simulink model "hierchical_control"  (R2023b)
settings: Solver=VariableStepAuto  StartTime=0.0  StopTime=tot_time  RelTol=1e-3
InitFcn:
  | addpath('TRAJECTORIES\');
  | %square_coplanar
  | circular_coplanar
StartFcn:
  | %% Setup Video e Timer
  | videoFile = 'Hierarchical_quad.avi';
  | %videoFile = 'Hierarchical_circ.avi';
  | videoObj = VideoWriter(videoFile);
  | videoObj.FrameRate = 30;
  | open(videoObj);
  | assignin('base','videoObj',videoObj);
  | 
  | 
  | t = timer('ExecutionMode','fixedSpacing','Period',0.05,'StartDelay',2,...
  |           'TimerFcn',@(~,~) captureFrame(findall(0,'Type','figure','Name','UAV Animation'), videoObj));
  | start(t);
  | 
  | 
  | assignin('base','videoTimer',t);
StopFcn:
  | % Default graphics settings
  | set(0, 'DefaultTextInterpreter', 'latex')
  | set(0, 'DefaultLegendInterpreter', 'latex')
  | set(0, 'DefaultAxesTickLabelInterpreter', 'latex')
  | lw = 2;
  | 
  | plot_errors = figure('Renderer', 'painters', 'Position', [10 10 900 650]);
  | 
  | subplot(2,1,1)
  | plot(out.tout, out.err_p.signals.values(1,:), 'k-', 'Linewidth', lw ,'Color', [0.2, 0.2, 0.2]);
  | hold on
  | plot(out.tout, out.err_p.signals.values(2,:), 'k-', 'Linewidth', lw ,'Color', [1, 0, 0]);
  | hold on
  | plot(out.tout, out.err_p.signals.values(3,:), 'k-', 'Linewidth', lw ,'Color', [0, 0, 1]);
  | 
  | legend({'x-axis', 'y-axis', 'z-axis'}, ...
  |        'Location', 'northeast', ...
  |        'Orientation', 'vertical', ...
  |        'FontSize', 16);
  | 
  | 
  | %xlabel('Time [s]')
  | ylabel('$e_p$ [m]')
  | 
  | set(gca, 'FontSize',20);
  | 
  | %Grid
  | grid on
  | box on
  | 
  | 
  | %----------------------------------------------------------
  | 
  | subplot(2,1,2)
  | plot(out.tout, out.dot_err_p.signals.values(1,:), 'k-', 'Linewidth', lw ,'Color', [0.2, 0.2, 0.2]);
  | hold on
  | plot(out.tout, out.dot_err_p.signals.values(2,:), 'k-', 'Linewidth', lw ,'Color', [1, 0, 0]);
  | hold on
  | plot(out.tout, out.dot_err_p.signals.values(3,:), 'k-', 'Linewidth', lw ,'Color', [0, 0, 1]);
  | 
  | legend({'x-axis', 'y-axis', 'z-axis'}, ...
  |        'Location', 'southeast', ...
  |        'Orientation', 'vertical', ...
  |        'FontSize', 16);
  | 
  | 
  | xlabel('Time [s]')
  | ylabel('$\dot{e}_p$ [m/s]')
  | 
  | set(gca, 'FontSize',20);
  | 
  | %Grid
  | grid on
  | box on
  | 
  | %Options
  | set(gcf,'color','w');
  | set(plot_errors, 'MenuBar', 'none', 'ToolBar', 'none');
  | 
  | exportgraphics(plot_errors, 'Hierarchical_lin_err.pdf');
  | 
  | %--------------------------------------------------
  | plot_errors_or = figure('Renderer', 'painters', 'Position', [10 10 900 650]);
  | 
  | subplot(2,1,1)
  | plot(out.tout, out.err_eta.signals.values(1,:), 'k-', 'Linewidth', lw ,'Color', [0.2, 0.2, 0.2]);
  | hold on
  | plot(out.tout, out.err_eta.signals.values(2,:), 'k-', 'Linewidth', lw ,'Color', [1, 0, 0]);
  | hold on
  | plot(out.tout, out.err_eta.signals.values(3,:), 'k-', 'Linewidth', lw ,'Color', [0, 0, 1]);
  | 
  | legend({'x-axis', 'y-axis', 'z-axis'}, ...
  |        'Location', 'southeast', ...
  |        'Orientation', 'vertical', ...
  |        'FontSize', 16);
  | 
  | 
  | ylabel('$e_{\eta}$ [rad]')
  | 
  | set(gca, 'FontSize',20);
  | 
  | %Grid
  | grid on
  | box on
  | 
  | 
  | %----------------------------------------------------------
  | 
  | subplot(2,1,2)
  | plot(out.tout, out.dot_err_eta.signals.values(1,:), 'k-', 'Linewidth', lw ,'Color', [0.2, 0.2, 0.2]);
  | hold on
  | plot(out.tout, out.dot_err_eta.signals.values(2,:), 'k-', 'Linewidth', lw ,'Color', [1, 0, 0]);
  | hold on
  | plot(out.tout, out.dot_err_eta.signals.values(3,:), 'k-', 'Linewidth', lw ,'Color', [0, 0, 1]);
  | 
  | legend({'x-axis', 'y-axis', 'z-axis'}, ...
  |        'Location', 'southeast', ...
  |        'Orientation', 'vertical', ...
  |        'FontSize', 16);
  | 
  | xlabel('Time [s]')
  | ylabel('$\dot{e_{\eta}}$ [rad/s]')
  | 
  | set(gca, 'FontSize',20);
  | 
  | %Grid
  | grid on
  | box on
  | 
  | %Options
  | set(gcf,'color','w');
  | set(plot_errors_or, 'MenuBar', 'none', 'ToolBar', 'none');
  | 
  | exportgraphics(plot_errors_or, 'Hierarchical_or_err.pdf');
  | 
  | 
  | %--------------------------------------------------------------
  | plot_pos_or = figure('Renderer', 'painters', 'Position', [10 10 900 650]);
  | 
  | subplot(2,1,1)
  | plot(out.tout, out.position.signals.values(1,:), 'k-', 'Linewidth', lw ,'Color', [0.2, 0.2, 0.2]);
  | hold on
  | plot(out.tout, out.position.signals.values(2,:), 'k-', 'Linewidth', lw ,'Color', [1, 0, 0]);
  | 
  | legend({'x-axis', 'y-axis'}, ...
  |        'Location', 'southeast', ...
  |        'Orientation', 'vertical', ...
  |        'FontSize', 16);
  | 
  | 
  | ylabel('$x,y$ [m]')
  | 
  | set(gca, 'FontSize',20);
  | 
  | %Grid
  | grid on
  | box on
  | 
  | 
  | %----------------------------------------------------------
  | 
  | subplot(2,1,2)
  | plot(out.tout, out.orientation.signals.values(1,:), 'k-', 'Linewidth', lw ,'Color', [0.2, 0.2, 0.2]);
  | hold on
  | plot(out.tout, out.orientation.signals.values(2,:), 'k-', 'Linewidth', lw ,'Color', [1, 0, 0]);
  | 
  | legend({'x-axis', 'y-axis'}, ...
  |        'Location', 'southeast', ...
  |        'Orientation', 'vertical', ...
  |        'FontSize', 16);
  | 
  | xlabel('Time [s]')
  | ylabel('$\phi,\theta$ [rad]')
  | 
  | set(gca, 'FontSize',20);
  | 
  | %Grid
  | grid on
  | box on
  | 
  | %Options
  | set(gcf,'color','w');
  | set(plot_pos_or, 'MenuBar', 'none', 'ToolBar', 'none');
  | 
  | exportgraphics(plot_pos_or, 'Hierarchical_pos_or.pdf');
  | 
  | %----------------------------------------------------------------------------------
  | 
  | plot_uT = figure('Renderer', 'painters', 'Position', [10 10 900 300]);
  | 
  | plot(out.tout, out.uT.signals.values, 'k-', 'Linewidth', lw ,'Color', [0.2, 0.2, 0.2]);
  | 
  | ylabel('$u_T$ [N]')
  | xlabel('Time [s]')
  | 
  | 
  | set(gca, 'FontSize',20);
  | 
  | %Grid
  | grid on
  | box on
  | 
  | %Options
  | set(gcf,'color','w');
  | set(plot_pos_or, 'MenuBar', 'none', 'ToolBar', 'none');
  | 
  | exportgraphics(plot_uT, 'Hierarchical_uT.pdf');
  | 
  | 
  | 
  | %---------------------------------------------------------------------
  | 
  | 
  | videoObj = evalin('base','videoObj');
  | t = evalin('base','videoTimer');
  | 
  | 
  | stop(t);
  | delete(t);
  | close(videoObj);
  | 
  | 
  | clear videoObj videoTimer
  | disp('Saved Video UAV');
undefined symbols (not defined in the file or in its folder): Ib, lin_vel_0, mass, Ts
libraries: robotcorelib x2, uavutilslib x1
settings Model: Creator=fabioruggiero  LastModifiedBy=laura
settings ModelReferenceCC: EnableRefExpFcnMdlSchedulingChecks=on

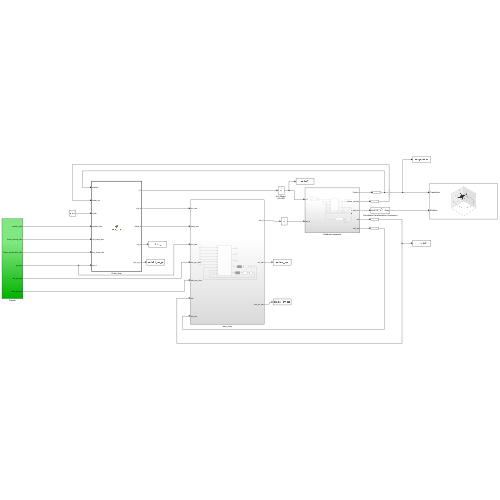
[thumbnail: Simulink's stored preview of the top-level diagram]
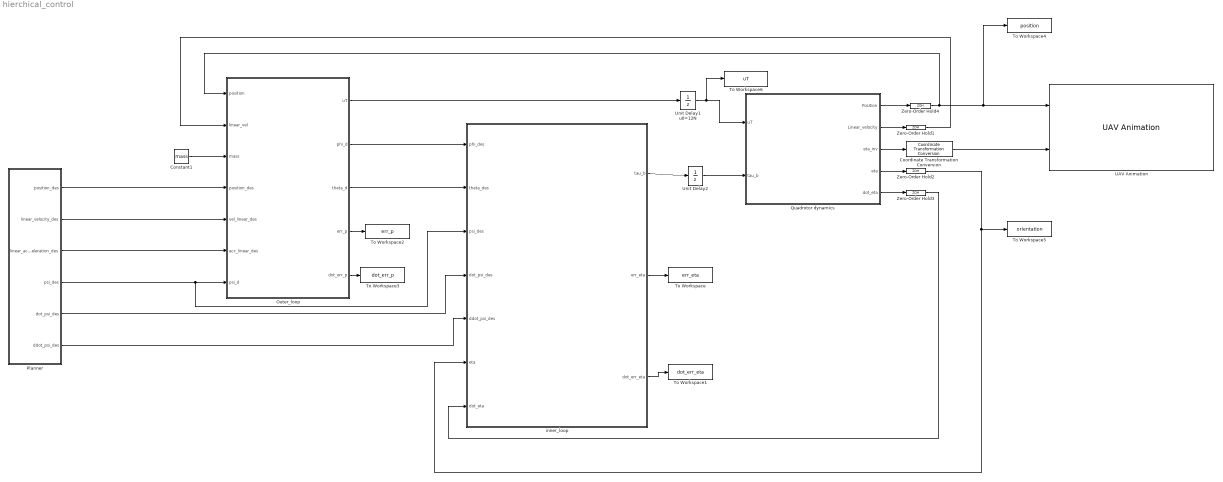
== system hierchical_control ==
  Constant1 : Constant  Value=mass
  Coordinate Transformation Conversion : robotcorelib/Coordinate Transformation Conversion  InputRepresentation=Euler Angles  InputEulerSequence=ZYX  ShowTrVecInputPort=on  OutputRepresentation=Quaternion  OutputEulerSequence=ZYX  ShowTrVecOutputPort=on  SimulateUsing=Interpreted execution
  Outer_loop : MATLAB Function  TreatAsAtomicUnit=on
  Planner : Subsystem
  Quadrotor dynamics : Subsystem
  To Workspace : ToWorkspace  VariableName=err_eta  SaveFormat=Structure With Time  SampleTime=-1
  To Workspace1 : ToWorkspace  VariableName=dot_err_eta  SaveFormat=Structure With Time  SampleTime=-1
  To Workspace2 : ToWorkspace  VariableName=err_p  SaveFormat=Structure With Time  SampleTime=-1
  To Workspace3 : ToWorkspace  VariableName=dot_err_p  SaveFormat=Structure With Time  SampleTime=-1
  To Workspace4 : ToWorkspace  VariableName=position  SaveFormat=Structure With Time  SampleTime=-1
  To Workspace5 : ToWorkspace  VariableName=orientation  SaveFormat=Structure With Time  SampleTime=-1
  To Workspace6 : ToWorkspace  VariableName=uT  SaveFormat=Structure With Time  SampleTime=-1
  UAV Animation : uavutilslib/UAV Animation  UAVType=Multirotor  UAVSize=1  InertialZDirection=Down  SampleTime=0.01
  Unit Delay1 u0=12N : UnitDelay  InitialCondition=12  SampleTime=Ts
  Unit Delay2 : UnitDelay  InitialCondition=[0 0 0]'  SampleTime=Ts
  Zero-Order Hold{1..4} (4 alike) : ZeroOrderHold  SampleTime=Ts
  inner_loop : Subsystem
  wires:
  Planner/1(position_des) -> Outer_loop/4(position_des)
  Planner/2(linear_velocity_des) -> Outer_loop/5(vel_linear_des)
  Planner/3(linear_acceleration_des) -> Outer_loop/6(acc_linear_des)
  Planner/4(psi_des) -> Outer_loop/7(psi_d), inner_loop/3(psi_des)
  Constant1/1 -> Outer_loop/3(mass)
  Planner/5(dot_psi_des) -> inner_loop/4(dot_psi_des)
  Planner/6(ddot_psi_des) -> inner_loop/5(ddot_psi_des)
  Outer_loop/1(uT) -> Unit Delay1 u0=12N/1
  Unit Delay1 u0=12N/1 -> To Workspace6/1, Quadrotor dynamics/1(uT)
  inner_loop/1(tau_b) -> Unit Delay2/1
  Unit Delay2/1 -> Quadrotor dynamics/2(tau_b)
  Quadrotor dynamics/1(Position) -> Zero-Order Hold4/1
  Quadrotor dynamics/2(Linear_velocity) -> Zero-Order Hold1/1
  Quadrotor dynamics/3(eta_inv) -> Coordinate Transformation Conversion/1
  Zero-Order Hold4/1 -> To Workspace4/1, UAV Animation/1, Outer_loop/1(position)
  Coordinate Transformation Conversion/1 -> UAV Animation/2
  Zero-Order Hold1/1 -> Outer_loop/2(linear_vel)
  inner_loop/2(err_eta) -> To Workspace/1
  inner_loop/3(dot_err_eta) -> To Workspace1/1
  Outer_loop/4(err_p) -> To Workspace2/1
  Outer_loop/5(dot_err_p) -> To Workspace3/1
  Quadrotor dynamics/5(dot_eta) -> Zero-Order Hold3/1
  Quadrotor dynamics/4(eta) -> Zero-Order Hold2/1
  Zero-Order Hold2/1 -> To Workspace5/1, inner_loop/6(eta)
  Zero-Order Hold3/1 -> inner_loop/7(dot_eta)
  Outer_loop/3(theta_d) -> inner_loop/2(theta_des)
  Outer_loop/2(phi_d) -> inner_loop/1(phi_des)

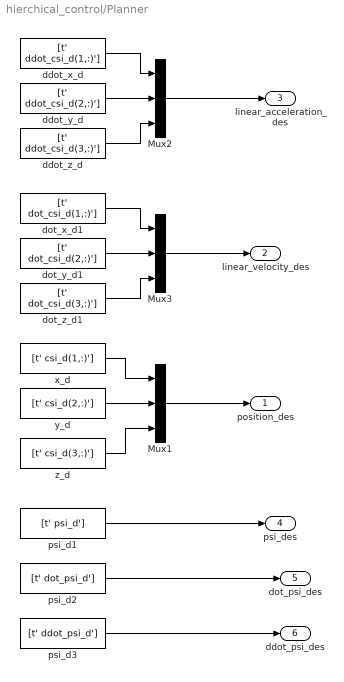
== system hierchical_control/Planner ==
  Mux1 : Mux  Inputs=3
  Mux2 : Mux  Inputs=3
  Mux3 : Mux  Inputs=3
  ddot_x_d : FromWorkspace  VariableName=[t' ddot_csi_d(1,:)']  SampleTime=Ts
  ddot_y_d : FromWorkspace  VariableName=[t' ddot_csi_d(2,:)']  SampleTime=Ts
  ddot_z_d : FromWorkspace  VariableName=[t' ddot_csi_d(3,:)']  SampleTime=Ts
  dot_x_d1 : FromWorkspace  VariableName=[t' dot_csi_d(1,:)']  SampleTime=Ts
  dot_y_d1 : FromWorkspace  VariableName=[t' dot_csi_d(2,:)']  SampleTime=Ts
  dot_z_d1 : FromWorkspace  VariableName=[t' dot_csi_d(3,:)']  SampleTime=Ts
  psi_d1 : FromWorkspace  VariableName=[t' psi_d']  SampleTime=Ts
  psi_d2 : FromWorkspace  VariableName=[t' dot_psi_d']  SampleTime=Ts
  psi_d3 : FromWorkspace  VariableName=[t' ddot_psi_d']  SampleTime=Ts
  x_d : FromWorkspace  VariableName=[t' csi_d(1,:)']  SampleTime=Ts
  y_d : FromWorkspace  VariableName=[t' csi_d(2,:)']  SampleTime=Ts
  z_d : FromWorkspace  VariableName=[t' csi_d(3,:)']  SampleTime=Ts
  position_des : Outport
  linear_velocity_des : Outport  Port=2
  linear_acceleration_des : Outport  Port=3
  psi_des : Outport  Port=4
  dot_psi_des : Outport  Port=5
  ddot_psi_des : Outport  Port=6
  wires:
  y_d/1 -> Mux1/2
  z_d/1 -> Mux1/3
  x_d/1 -> Mux1/1
  ddot_y_d/1 -> Mux2/2
  ddot_z_d/1 -> Mux2/3
  ddot_x_d/1 -> Mux2/1
  Mux2/1 -> linear_acceleration_des/1
  Mux1/1 -> position_des/1
  dot_y_d1/1 -> Mux3/2
  dot_z_d1/1 -> Mux3/3
  dot_x_d1/1 -> Mux3/1
  Mux3/1 -> linear_velocity_des/1
  psi_d1/1 -> psi_des/1
  psi_d3/1 -> ddot_psi_des/1
  psi_d2/1 -> dot_psi_des/1

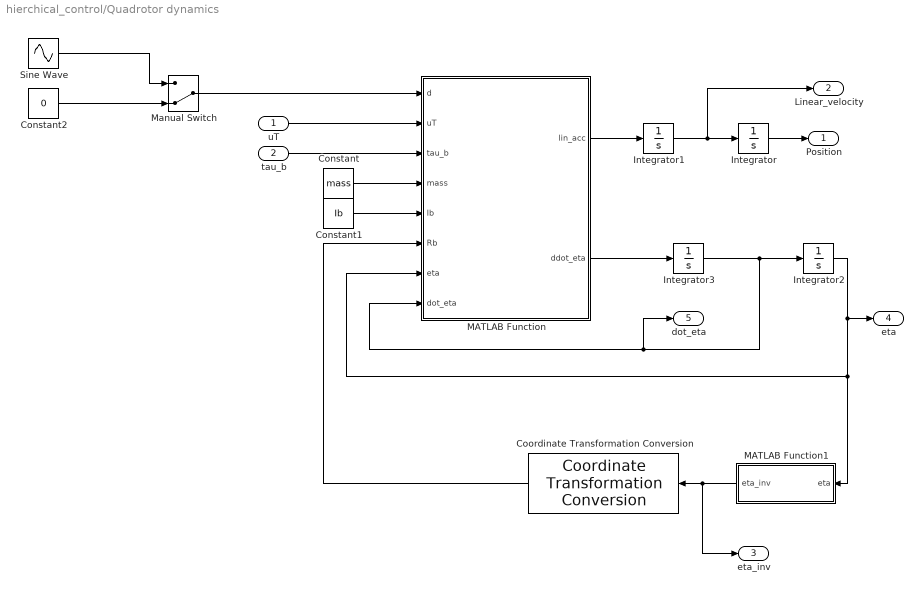
== system hierchical_control/Quadrotor dynamics ==
  uT : Inport
  tau_b : Inport  Port=2
  Constant : Constant  Value=mass
  Constant1 : Constant  Value=Ib
  Constant2 : Constant  Value=0
  Coordinate Transformation Conversion : robotcorelib/Coordinate Transformation Conversion  InputRepresentation=Euler Angles  InputEulerSequence=ZYX  ShowTrVecInputPort=on  OutputRepresentation=Rotation Matrix  OutputEulerSequence=ZYX  ShowTrVecOutputPort=on  SimulateUsing=Interpreted execution
  Integrator : Integrator  InitialCondition=[0 0 -1]'
  Integrator1 : Integrator  InitialCondition=lin_vel_0'
  Integrator2 : Integrator  InitialCondition=[0,0,0]'
  Integrator3 : Integrator  InitialCondition=[0 0 0]'
  MATLAB Function : MATLAB Function  TreatAsAtomicUnit=on
  MATLAB Function1 : MATLAB Function  TreatAsAtomicUnit=on
  Manual Switch : ManualSwitch  CurrentSetting=0
  Sine Wave : Sin  Frequency=0.2  SampleTime=0
  Position : Outport
  Linear_velocity : Outport  Port=2
  eta_inv : Outport  Port=3
  eta : Outport  Port=4
  dot_eta : Outport  Port=5
  wires:
  tau_b/1 -> MATLAB Function/3(tau_b)
  Integrator/1 -> Position/1
  MATLAB Function/1(lin_acc) -> Integrator1/1
  uT/1 -> MATLAB Function/2(uT)
  Integrator1/1 -> Integrator/1, Linear_velocity/1
  Integrator3/1 -> Integrator2/1, dot_eta/1, MATLAB Function/8(dot_eta)
  MATLAB Function/2(ddot_eta) -> Integrator3/1
  Constant/1 -> MATLAB Function/4(mass)
  Constant1/1 -> MATLAB Function/5(Ib)
  Integrator2/1 -> MATLAB Function1/1(eta), MATLAB Function/7(eta), eta/1
  MATLAB Function1/1(eta_inv) -> eta_inv/1, Coordinate Transformation Conversion/1
  Coordinate Transformation Conversion/1 -> MATLAB Function/6(Rb)
  Sine Wave/1 -> Manual Switch/1
  Constant2/1 -> Manual Switch/2
  Manual Switch/1 -> MATLAB Function/1(d)

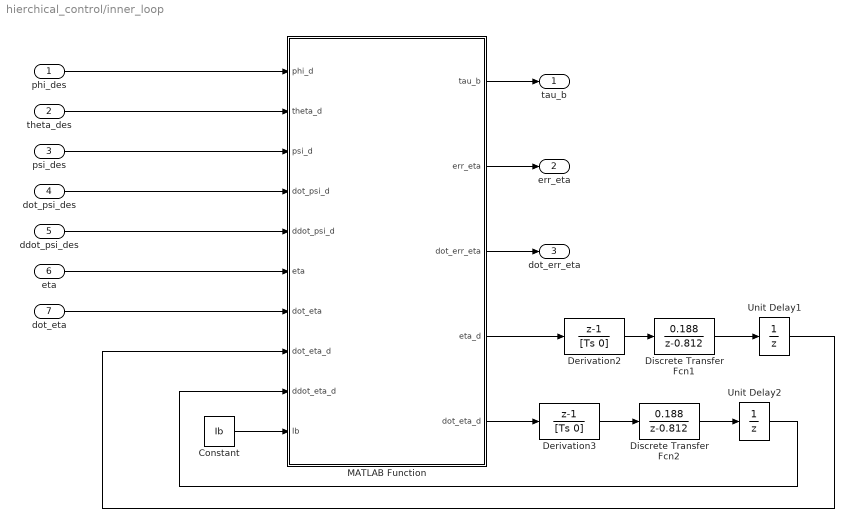
== system hierchical_control/inner_loop ==
  phi_des : Inport
  theta_des : Inport  Port=2
  psi_des : Inport  Port=3
  dot_psi_des : Inport  Port=4
  ddot_psi_des : Inport  Port=5
  eta : Inport  Port=6
  dot_eta : Inport  Port=7
  Constant : Constant  Value=Ib
  Derivation2 : DiscreteTransferFcn  Numerator=[1 -1]  Denominator=[Ts 0]  InitialStates=[0 0 0]'  SampleTime=Ts
  Derivation3 : DiscreteTransferFcn  Numerator=[1 -1]  Denominator=[Ts 0]  InitialStates=[0 0 0]'  SampleTime=Ts
  Discrete Transfer Fcn1 : DiscreteTransferFcn  Numerator=0.188  Denominator=[1 -0.812]
  Discrete Transfer Fcn2 : DiscreteTransferFcn  Numerator=0.188  Denominator=[1 -0.812]
  MATLAB Function : MATLAB Function  TreatAsAtomicUnit=on
  Unit Delay1 : UnitDelay  InitialCondition=[0 0 0]'  SampleTime=Ts
  Unit Delay2 : UnitDelay  InitialCondition=[0 0 0]'  SampleTime=Ts
  tau_b : Outport
  err_eta : Outport  Port=2
  dot_err_eta : Outport  Port=3
  wires:
  theta_des/1 -> MATLAB Function/2(theta_d)
  phi_des/1 -> MATLAB Function/1(phi_d)
  psi_des/1 -> MATLAB Function/3(psi_d)
  Constant/1 -> MATLAB Function/10(Ib)
  dot_psi_des/1 -> MATLAB Function/4(dot_psi_d)
  ddot_psi_des/1 -> MATLAB Function/5(ddot_psi_d)
  Derivation2/1 -> Discrete Transfer Fcn1/1
  MATLAB Function/4(eta_d) -> Derivation2/1
  Unit Delay1/1 -> MATLAB Function/8("dot_eta_d ")
  Derivation3/1 -> Discrete Transfer Fcn2/1
  Unit Delay2/1 -> MATLAB Function/9(ddot_eta_d)
  MATLAB Function/1(tau_b) -> tau_b/1
  MATLAB Function/2(err_eta) -> err_eta/1
  MATLAB Function/3(dot_err_eta) -> dot_err_eta/1
  eta/1 -> MATLAB Function/6(eta)
  dot_eta/1 -> MATLAB Function/7(dot_eta)
  Discrete Transfer Fcn2/1 -> Unit Delay2/1
  Discrete Transfer Fcn1/1 -> Unit Delay1/1
  MATLAB Function/5(dot_eta_d) -> Derivation3/1

== matlab function hierchical_control/Outer_loop ==
  data: uT output; phi_d output; theta_d output; position input; err_p output; linear_vel input; mass input; position_des input; vel_linear_des input; acc_linear_des input; psi_d input; dot_err_p output
function [ uT, phi_d, theta_d, err_p, dot_err_p] = outer_loop( position, linear_vel, mass, ...
    position_des, vel_linear_des, acc_linear_des,psi_d)

    %Linear gain matrix
    K_p = [10 0 0 sqrt(10) 0 0;
           0 10 0 0 sqrt(10) 0;
           0 0 10 0 0 sqrt(10)];
    g = 9.81;
    
    %Compute the position error
    err_p = position - position_des;
    
    %Compute the time derivative of the position error
    dot_err_p = linear_vel - vel_linear_des;
    
    mu_d = (-K_p*[err_p' dot_err_p']'+ acc_linear_des);
    
    %mu_d(3) must be less than g (in module)
    mu_d(3) = max(min(mu_d(3), 0.9*g), -0.9*g);
    
    %Compute the commanded total thrust
    uT = mass*sqrt(mu_d(1)^2 + mu_d(2)^2 + (mu_d(3)-g)^2);
    
    %Compute the desired phi
    phi_d = asin((mass/uT)*(mu_d(2)*cos(psi_d)-mu_d(1)*sin(psi_d)));
    
    %Compute the desired theta
    theta_d = atan((mu_d(1)*cos(psi_d)+mu_d(2)*sin(psi_d))/(mu_d(3)-g));

end

== matlab function hierchical_control/inner_loop/MATLAB Function ==
  data: tau_b output; phi_d input; theta_d input; psi_d input; dot_psi_d input; ddot_psi_d input; eta input; dot_eta input; dot_eta_d input; ddot_eta_d input; Ib input; err_eta output; dot_err_eta output; eta_d output; dot_eta_d output
function [ tau_b, err_eta, dot_err_eta, eta_d , dot_eta_d] = fcn(phi_d,theta_d, psi_d, dot_psi_d, ddot_psi_d, eta, dot_eta, dot_eta_d, ddot_eta_d, Ib)

%% WRITE HERE THE INNER-LOOP CONTROL
% zb_des: desired z-axis of the body frame
% Rb: current rotation matrix
% dot_Rb_des: time-derivative of the desired rotation matrix
% omega_bb: current angular velocity expressed in the body frame
% dot_omega_bb_des: desired angular acceleration expressed in the body
% frame
% xb_des: desired x-axis of the body frame form the planner
% Ib: inertia matrix of the UAV with respect to the body frame
% ---
% Rb_des: desired rotation matrix
% omega_bb_des: desired angular velocity expressed in the body frame (given
% below as a hint)
% tau: commanded control torque
% err_R: rotational error in SO(3)
% err_W: angular velocity error in SO(3)

%Angular gain matrix
Ke = [150 0 0 sqrt(150) 0 0; 
      0 150 0 0 sqrt(150) 0;
      0 0 150 0 0 sqrt(150)];

%Desired orientation 
eta_d = [phi_d theta_d psi_d]';

% We replace the derivative values computed numerically with those provided by the trajectory planner, which are more accurate and not affected by numerical differentiation errors.
dot_eta_d(3) = dot_psi_d;
ddot_eta_d(3) = ddot_psi_d;

%Compute the orientation errors
err_eta = eta-eta_d;
dot_err_eta = dot_eta-dot_eta_d;

Q = [1 0 -sin(eta(2));0 cos(eta(1)) cos(eta(2))*sin(eta(1));0 -sin(eta(1)) cos(eta(1))*cos(eta(2))];

Q_dot = [0 , 0 , -cos(eta(2))*dot_eta(2) ;
             0 , -sin(eta(1))*dot_eta(1) , cos(eta(1))*cos(eta(2))*dot_eta(1)-sin(eta(1))*sin(eta(2))*dot_eta(2) ;
             0 , -cos(eta(1))*dot_eta(1) , -sin(eta(1))*cos(eta(2))*dot_eta(1)-sin(eta(2))*cos(eta(1))*dot_eta(2)];

C = Q'*skew(Q*dot_eta)*Ib*Q + Q'*Ib*Q_dot;

%Compute virtual input for the feedback linearization
tau_tilde = -Ke*[err_eta' dot_err_eta']' + ddot_eta_d;

% Check on theta for singularities in Q
epsilon = 1e-4;
if abs(eta(2) - pi/2) < epsilon
    eta(2) = eta(2) - sign(eta(2)) * epsilon;
end

%Compute the commanded control torque
tau_b = Ib*Q*tau_tilde+ inv(Q)'*C*dot_eta;

end

function S = skew(v)
if(numel(v)~= 1)
S= [0 -v(3) v(2); 
    v(3) 0 -v(1);
    -v(2) v(1) 0];
else
S= zeros(3);
end
end

== matlab function hierchical_control/Quadrotor dynamics/MATLAB Function1 ==
  data: eta input; eta_inv output
function eta_inv = fcn(eta)

eta_inv = [eta(3) eta(2) eta(1)]';

== matlab function hierchical_control/Quadrotor dynamics/MATLAB Function ==
  data: d input; uT input; lin_acc output; tau_b input; mass input; Ib input; Rb input; eta input; dot_eta input; ddot_eta output
function [lin_acc,ddot_eta] = fcn(d,uT,tau_b,mass, Ib ,Rb, eta, dot_eta)

    lin_acc = 9.81*[0 0 1]'-(uT/mass)*Rb*[0 0 1]'+d*ones(3,1);
    
    
    Q = [1 0 -sin(eta(2));0 cos(eta(1)) cos(eta(2))*sin(eta(1));0 -sin(eta(1)) cos(eta(1))*cos(eta(2))];
    Q_dot = [0 , 0 , -cos(eta(2))*dot_eta(2) ;
                 0 , -sin(eta(1))*dot_eta(1) , cos(eta(1))*cos(eta(2))*dot_eta(1)-sin(eta(1))*sin(eta(2))*dot_eta(2) ;
                 0 , -cos(eta(1))*dot_eta(1) , -sin(eta(1))*cos(eta(2))*dot_eta(1)-sin(eta(2))*cos(eta(1))*dot_eta(2)];
    C = Q'*skew(Q*dot_eta)*Ib*Q + Q'*Ib*Q_dot;
    M = Q'*Ib*Q;
    
    ddot_eta = M\(-C*dot_eta + Q'*tau_b);

end


function S = skew(v)
if(numel(v)~= 1)
S= [0 -v(3) v(2); 
    v(3) 0 -v(1);
    -v(2) v(1) 0];
else
S= zeros(3);
end
end
